simulink model "Q5"  (R2016a)
settings: Solver=VariableStepAuto  StartTime=0.0  StopTime=10.0  RelTol=1e-3
settings Model: Creator=negfir  LastModifiedBy=negfir

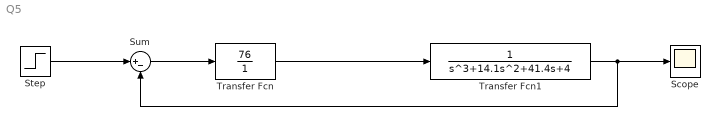
== system Q5 ==
  Scope : Scope
  Step : Step  After=100  SampleTime=0
  Sum : Sum  Inputs=|+-
  Transfer Fcn : TransferFcn  Numerator=[76]  Denominator=[1]
  Transfer Fcn1 : TransferFcn  Denominator=[1 14.1 41.4 4]
  wires:
  Transfer Fcn/1 -> Transfer Fcn1/1
  Step/1 -> Sum/1
  Sum/1 -> Transfer Fcn/1
  Transfer Fcn1/1 -> Scope/1, Sum/2
